simulink model "on_off_keying"  (R2018a)
settings: Solver=VariableStepAuto  StartTime=0.0  StopTime=10  RelTol=1e-3
libraries: commrandsrc3 x1
settings Model: Creator=hp  LastModifiedBy=hp

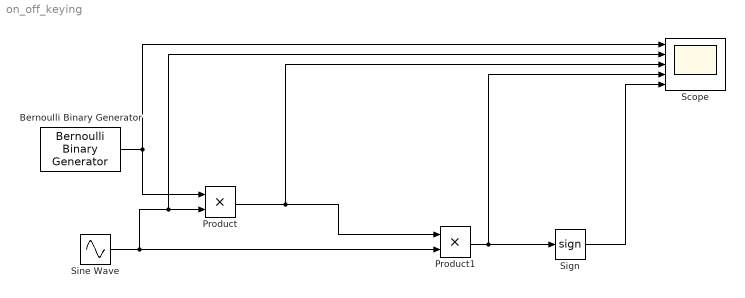
== system on_off_keying ==
  Bernoulli Binary Generator : commrandsrc3/Bernoulli Binary Generator  ProbabilityOfZero=0.4  SeedSource=Auto  Seed=0  SampleTime=1  SamplesPerFrame=1  OutputDataType=double  SimulateUsing=Interpreted execution
  Product : Product
  Product1 : Product
  Scope : Scope  NumInputPorts=5
  Sign : Signum
  Sine Wave : Sin  SampleTime=0.001
  wires:
  Bernoulli Binary Generator/1 -> Scope/1, Product/1
  Product1/1 -> Scope/4, Sign/1
  Sine Wave/1 -> Product1/2, Scope/2, Product/2
  Product/1 -> Scope/3, Product1/1
  Sign/1 -> Scope/5
